simulink model "simulacao_ss_compatibilidade"  (Simulink 7.2)
settings: Solver=ode3  SolverMode=SingleTasking  StartTime=0.0  StopTime=10.0  FixedStep=0.0001  RelTol=1e-3
values from neighbouring files (symbols this model uses):
  Ki = Kext(3)    [MDLsspace.m]    (also in dadosSS.mat = -0.0370352066606; ssGera.m)
  Kproc = [Kext(1), Kext(2)]    [MDLsspace.m]    (also in dadosSS.mat = [-0.861797620241 -0.503028275301]; ssGera.m)
  L = (acker(A', C', polosObs))'    [MDLsspace.m]    (also in dadosSS.mat = [-0.306409103952 0.415866033676]; ssGera.m)
settings Model: Creator=root  LastModifiedBy=aluno  CovMetricSettings=dwe  CovHtmlReporting=off  covSaveCumulativeToWorkspaceVar=off  CovSaveSingleToWorkspaceVar=off
settings SolverCC: ZeroCrossAlgorithm=Adaptive
settings DataIOCC: LimitDataPoints=off  SaveFormat=StructureWithTime
settings OptimizationCC: ExpressionDepthLimit=128
settings DebuggingCC: UnderspecifiedInitializationDetection=Simplified  MergeDetectMultiDrivingBlocksExec=error  MaxConsecutiveZCsMsg=none  SolverPrmCheckMsg=none  FcnCallInpInsideContextMsg=Enable All  StateNameClashWarn=none  StrictBusMsg=ErrorLevel1
settings HardwareCC: ProdIntDivRoundTo=Zero  ProdEndianess=LittleEndian  ProdHWDeviceType=Specified
settings CodeAppCC: CustomSymbolStrType=$N$R$M_T
settings GRTTargetCC: TargetFunctionLibrary=C99 (ISO)

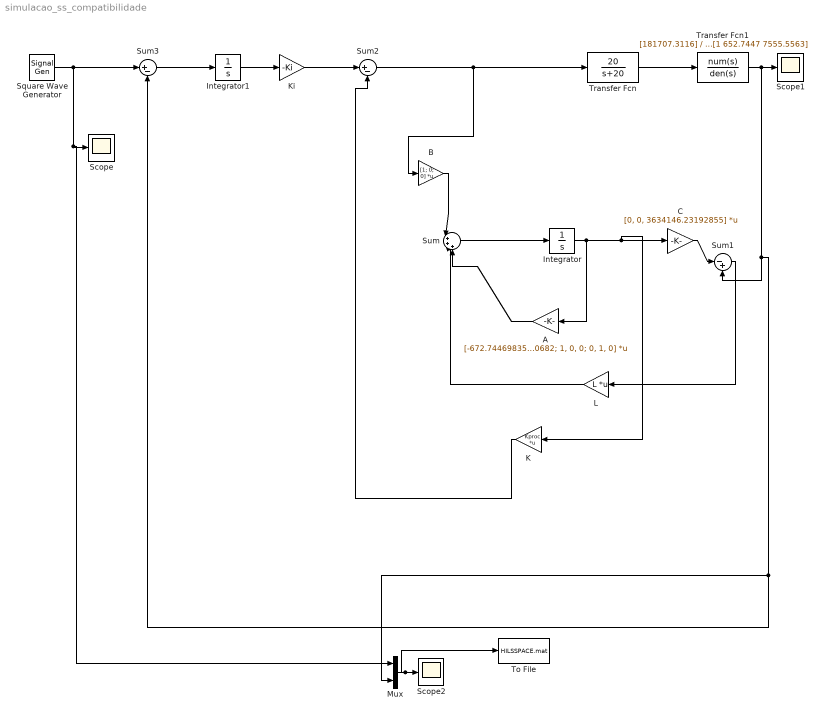
== system simulacao_ss_compatibilidade ==
  A : Gain  Orientation=left  Gain="[-672.744698351479,  -20610.4503165634, -151111.126990682; 1, 0, 0; 0, 1, 0]"  Multiplication=Matrix(K*u)
  B : Gain  Gain=[1; 0; 0]  Multiplication=Matrix(K*u)
  C : Gain  Gain=[0, 0, 3634146.23192855]  Multiplication=Matrix(K*u)
  Integrator : Integrator
  Integrator1 : Integrator
  K : Gain  Orientation=left  Gain=Kproc  Multiplication=Matrix(K*u)
  Ki : Gain  Gain=-Ki
  L : Gain  Orientation=left  Gain=L  Multiplication=Matrix(K*u)
  Mux : Mux  Inputs=2
  Scope : Scope
      settings: YMin=-56.25  YMax=56.25
  Scope1 : Scope
      settings: YMin=-56.25  YMax=56.25
  Scope2 : Scope
      settings: YMin=-56.25  YMax=56.25
  Square Wave Generator : SignalGenerator  WaveForm=square  Amplitude=45  Units=rad/sec
  Sum : Sum  Inputs=|+++
  Sum1 : Sum  Inputs=|-+
  Sum2 : Sum  Inputs=|+-
  Sum3 : Sum  Inputs=|+-
  To File : ToFile  Filename=HILSSPACE.mat
  Transfer Fcn : TransferFcn  Numerator=[20]  Denominator=[1, 20]
  Transfer Fcn1 : TransferFcn  Numerator=[181707.3116]  Denominator=[1 652.7447 7555.5563]
  wires:
  Sum2/1 -> B/1, Transfer Fcn/1
  Sum/1 -> Integrator/1
  Integrator/1 -> A/1, C/1, K/1
  A/1 -> Sum/3
  C/1 -> Sum1/1
  B/1 -> Sum/1
  Sum1/1 -> L/1
  L/1 -> Sum/2
  Integrator1/1 -> Ki/1
  Ki/1 -> Sum2/1
  Transfer Fcn1/1 -> Scope1/1, Mux/2, Sum3/2, Sum1/2
  Sum3/1 -> Integrator1/1
  Square Wave Generator/1 -> Mux/1, Scope/1, Sum3/1
  Transfer Fcn/1 -> Transfer Fcn1/1
  Mux/1 -> Scope2/1, To File/1
  K/1 -> Sum2/2
